simulink model "Subsystem"  (R2020b)
settings: Solver=VariableStepAuto  StartTime=0.0  StopTime=10.0  RelTol=1e-3
model workspace (MAT data in the model file):
  b1 = 350
  b2 = 15020
  k1 = 80000
  k2 = 500000
  m1 = 2500
  m2 = 320
settings Model: Creator=varunraj  LastModifiedBy=varunraj
settings DataIOCC: SaveOutput=off  SaveTime=off

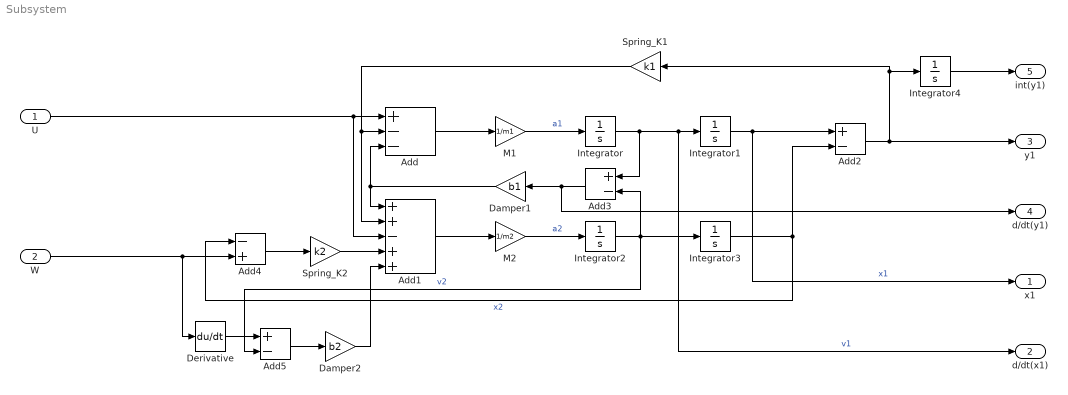
== system Subsystem ==
  U : Inport  OutDataTypeStr=double  PortDimensions=1  SampleTime=0
  W : Inport  Port=2  OutDataTypeStr=double  PortDimensions=1  SampleTime=0
  Add : Sum  Inputs=+--
  Add1 : Sum  Inputs=++-++
  Add2 : Sum  Inputs=+-
  Add3 : Sum  Inputs=+-
  Add4 : Sum  Inputs=-+
  Add5 : Sum  Inputs=+-
  Damper1 : Gain  Gain=b1
  Damper2 : Gain  Gain=b2
  Derivative : Derivative
  Integrator{,1..4} (5 alike) : Integrator
  M1 : Gain  Gain=1/m1
  M2 : Gain  Gain=1/m2
  Spring_K1 : Gain  Gain=k1
  Spring_K2 : Gain  Gain=k2
  x1 : Outport  OutDataTypeStr=double  PortDimensions=1  SampleTime=0
  d/dt(x1) : Outport  Port=2  OutDataTypeStr=double  PortDimensions=1  SampleTime=0
  y1 : Outport  Port=3  OutDataTypeStr=double  PortDimensions=1  SampleTime=0
  d/dt(y1) : Outport  Port=4  OutDataTypeStr=double  PortDimensions=1  SampleTime=0
  int(y1) : Outport  Port=5  OutDataTypeStr=double  PortDimensions=1  SampleTime=0
  wires:
  Add5/1 -> Damper2/1
  Damper1/1 -> Add/3, Add1/1
  Integrator3/1 -> Add2/2, Add4/1  "x2"
  M2/1 -> Integrator2/1  "a2"
  Integrator4/1 -> int(y1)/1
  W/1 -> Add4/2, Derivative/1
  M1/1 -> Integrator/1  "a1"
  Integrator2/1 -> Integrator3/1, Add3/2, Add5/2  "v2"
  Add1/1 -> M2/1
  Spring_K2/1 -> Add1/4
  Integrator/1 -> Integrator1/1, d/dt(x1)/1, Add3/1  "v1"
  Add2/1 -> Integrator4/1, Spring_K1/1, y1/1
  Spring_K1/1 -> Add/2, Add1/2
  Integrator1/1 -> Add2/1, x1/1  "x1"
  U/1 -> Add/1, Add1/3
  Add4/1 -> Spring_K2/1
  Add/1 -> M1/1
  Add3/1 -> Damper1/1, d/dt(y1)/1
  Derivative/1 -> Add5/1
  Damper2/1 -> Add1/5
